simulink model "levitron_ctrl"  (Simulink 7.1)
settings: Solver=ode45  StartTime=0.0  StopTime=10.0  RelTol=1e-3
settings Model: Creator=volgy  LastModifiedBy=volgy

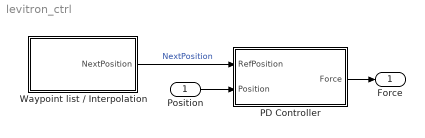
== system levitron_ctrl ==
  Position : Inport  PortDimensions=1  DataType=single  OutDataType=sfix(16)  OutScaling=2^0  OutDataTypeStr=single
  PD Controller : Subsystem  AncestorBlock=levitron_lib/PD Controller
  Waypoint list / Interpolation : Subsystem  AncestorBlock=levitron_lib/Waypoint list // Interpolation  mask{sample_time=0.2, time_values=[0 20 40 60 80 100], output_values=[10 50 30 20 40 10]}
      mask prompts: sample_time "Sample Time (s)"; time_values "Time Values"; output_values "Output Values"
  Force : Outport  PortDimensions=1  DataType=single  OutDataType=sfix(16)  OutScaling=2^0  OutDataTypeStr=single
  wires:
  Waypoint list / Interpolation/1(NextPosition) -> PD Controller/1(RefPosition)  "NextPosition"
  Position/1 -> PD Controller/2(Position)
  PD Controller/1(Force) -> Force/1

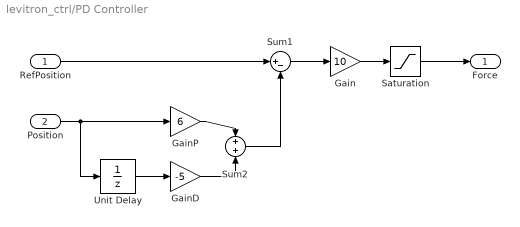
== system levitron_ctrl/PD Controller ==
  RefPosition : Inport
  Position : Inport  Port=2
  Gain : Gain  Gain=10  ParameterDataType=sfix(16)  ParameterScaling=2^0  OutDataType=sfix(16)  OutScaling=2^0
  GainD : Gain  Gain=-5  ParameterDataType=sfix(16)  ParameterScaling=2^0  OutDataType=sfix(16)  OutScaling=2^0
  GainP : Gain  Gain=6  ParameterDataType=sfix(16)  ParameterScaling=2^0  OutDataType=sfix(16)  OutScaling=2^0
  Saturation : Saturate  UpperLimit=100  LowerLimit=0  OutDataType=sfix(16)  OutScaling=2^0
  Sum1 : Sum  Inputs=|+-  OutDataType=sfix(16)  OutScaling=2^0
  Sum2 : Sum  Inputs=+|+  OutDataType=sfix(16)  OutScaling=2^0
  Unit Delay : UnitDelay  X0=10  SampleTime=-1
  Force : Outport
  wires:
  Unit Delay/1 -> GainD/1
  GainP/1 -> Sum2/1
  GainD/1 -> Sum2/2
  Sum1/1 -> Gain/1
  Gain/1 -> Saturation/1
  Saturation/1 -> Force/1
  RefPosition/1 -> Sum1/1
  Position/1 -> GainP/1, Unit Delay/1
  Sum2/1 -> Sum1/2

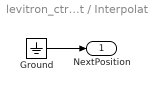
== system levitron_ctrl/Waypoint list / Interpolation ==
  Ground : Ground
  NextPosition : Outport  PortDimensions=1  DataType=single  OutDataTypeStr=single
  wires:
  Ground/1 -> NextPosition/1
